simulink model "planemodel"  (Simulink 3.00)
settings: Solver=ode15s  SolverMode=SingleTasking  StartTime=0.0  StopTime=10  MaxStep=0.1  RelTol=1e-3  AbsTol=1e-3
values from neighbouring files (symbols this model uses):
  Kf = 1.27*[1 1]    [design4.m]
  T_f = 0.28    [design4.m]
undefined symbols (not defined in the file or in its folder): A, B, C, Ctheta, D
libraries: pilotlib x1
settings Model: SaveTime=off  SaveOutput=off  RTWTemplateMakefile=grt_unix.tmf  Creator=sven  LastModifiedBy=sven

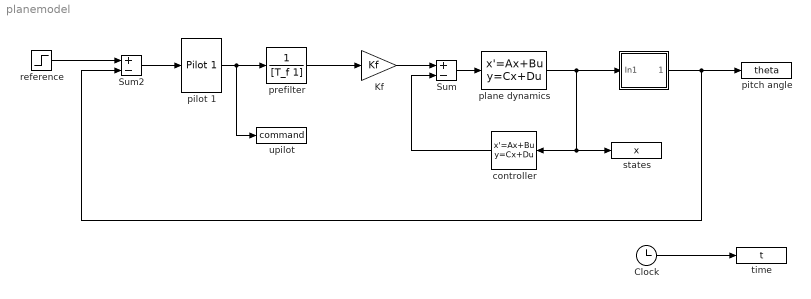
== system planemodel ==
  " " : Subsystem  mask(Matrix Gain){K=Ctheta}
      mask prompts: K "Gain matrix:"
      mask help: Matrix Gain.
      mask Help: Multiplies input vector by entered matrix to produce output vector (y=Au).
      mask Display: disp('Ctheta')
  Clock : Clock
      settings: DisplayTime=off  Decimation=10
  Kf : Gain  Gain=Kf  SaturateOnIntegerOverflow=on
  Sum : Sum  Inputs=+-  SaturateOnIntegerOverflow=on
  Sum2 : Sum  Inputs=+-  SaturateOnIntegerOverflow=on
  controller : StateSpace  Orientation=left  A=[]  B=[]  C=[]  D=K  X0=0  mask(Matrix gain){@1=L}
      mask prompts: @1 "Gain matrix:"
      mask help: Matrix Gain:
      mask init:
      | K = @1;
      mask Help: Multiplies input vector by entered matrix to produce output vector.
      mask Display: disp('L')
  pilot 1 : pilotlib/Pilot 1
  pitch angle : ToWorkspace  VariableName=theta  SampleTime=0  SaveFormat=Matrix
      settings: Buffer=10000
  plane dynamics : StateSpace  A=A  B=B  C=C  D=D  X0=0
  prefilter : TransferFcn  Numerator=[1]  Denominator=[T_f 1]
  reference : Step  Time=0  Before=0  After=1  SampleTime=0
  states : ToWorkspace  VariableName=x  SampleTime=0  SaveFormat=Matrix
      settings: Buffer=10000
  time : ToWorkspace  VariableName=t  SampleTime=0  SaveFormat=Matrix
      settings: Buffer=10000
  upilot : ToWorkspace  VariableName=command  SampleTime=0  SaveFormat=Matrix
      settings: Buffer=10000
  wires:
  " "/1(Out1) -> Sum2/2, pitch angle/1
  Sum2/1 -> pilot 1/1
  reference/1 -> Sum2/1
  plane dynamics/1 -> " "/1(In1), controller/1, states/1
  prefilter/1 -> Kf/1
  Sum/1 -> plane dynamics/1
  controller/1 -> Sum/2
  Kf/1 -> Sum/1
  pilot 1/1 -> prefilter/1, upilot/1
  Clock/1 -> time/1

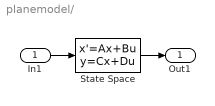
== system planemodel/  ==
  In1 : Inport  Port=1  PortWidth=-1  SampleTime=-1  DataType=auto
      settings: SignalType=auto
  State Space : StateSpace  A=[]  B=[]  C=[]  D=K  X0=0
  Out1 : Outport  Port=1
  wires:
  In1/1 -> State Space/1
  State Space/1 -> Out1/1
